simulink model "simulink_test_bt"  (R2024a)
settings: Solver=ode15s  StartTime=0.0  StopTime=10.0  RelTol=1e-3
values from neighbouring files (symbols this model uses):
  r1 = BodyTree(J, B)    [class_test_hybrid.m]    (also in fd_mex_test.m = BodyTree(J1, B1); methods_test.m = BodyTree(J1, B1); test_bodyjacobian.m = BodyTree(J1, B1); test_kinematics.m = BodyTree(J1, B1))
libraries: SoftRobotics x1
settings Model: Creator=pietro  LastModifiedBy=pietro
settings RTWCC: GenerateReport=on  GPUComputeCapability=3.5

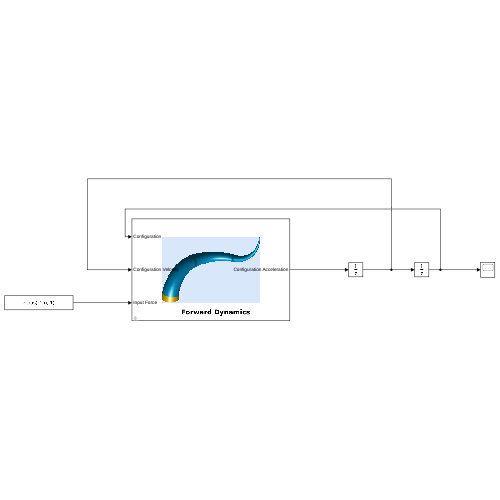
[thumbnail: Simulink's stored preview of the top-level diagram]
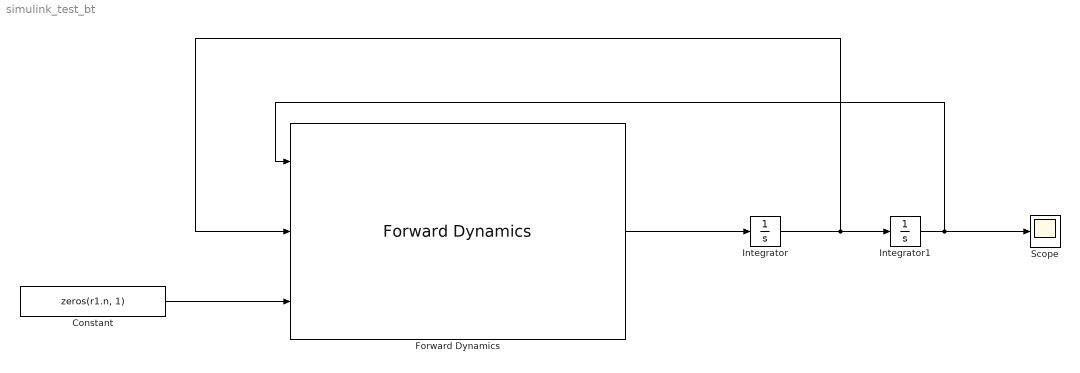
== system simulink_test_bt ==
  Constant : Constant  Value=zeros(r1.n, 1)
  Forward Dynamics : SoftRobotics/Forward Dynamics  RobotModel=r1  SimulateUsing=Code generation
      settings: SourceProductName=Jelly
  Integrator : Integrator
  Integrator1 : Integrator  InitialCondition=ones(r1.n, 1)
  Scope : Scope
  wires:
  Forward Dynamics/1 -> Integrator/1
  Integrator/1 -> Forward Dynamics/2, Integrator1/1
  Constant/1 -> Forward Dynamics/3
  Integrator1/1 -> Forward Dynamics/1, Scope/1
